simulink library "ITKLib"  (R2022b)
settings: Solver=FixedStepDiscrete  StartTime=0.0  StopTime=10.0  FixedStep=0.01  RelTol=1e-3  EnableMultiTasking=on
values from neighbouring files (symbols this model uses):
  Glb_WhlRollgRd_SC = single(0.36)    [init_Global.m]
undefined symbols (not defined in the file or in its folder): docblock, SlDemoSign, SlDemoSign_Positive_SC, TaskTime_100ms_SC, TaskTime_10ms_SC, VehRefSpd_vMaxRefSpd_C
libraries: simulink x51, $bdroot x45, ITKLib_V14 x1
(part 7 of 10)

== system ITKLib/BitOperation/Subsystem2 ==
  Pos : Inport
  In : Inport  Port=2  OutDataTypeStr=uint8
  Bitwise Operator : simulink/Logic and Bit Operations/Bitwise Operator  logicop=OR  UseBitMask=on  BitMask=bin2dec('00000001')  BitMaskRealWorld=Stored Integer
  Bitwise Operator10 : simulink/Logic and Bit Operations/Bitwise Operator  logicop=OR  UseBitMask=on  BitMask=bin2dec('00100000')  BitMaskRealWorld=Stored Integer
  Bitwise Operator12 : simulink/Logic and Bit Operations/Bitwise Operator  logicop=OR  UseBitMask=on  BitMask=bin2dec('01000000')  BitMaskRealWorld=Stored Integer
  Bitwise Operator14 : simulink/Logic and Bit Operations/Bitwise Operator  logicop=OR  UseBitMask=on  BitMask=bin2dec('10000000')  BitMaskRealWorld=Stored Integer
  Bitwise Operator2 : simulink/Logic and Bit Operations/Bitwise Operator  logicop=OR  UseBitMask=on  BitMask=bin2dec('00000010')  BitMaskRealWorld=Stored Integer
  Bitwise Operator4 : simulink/Logic and Bit Operations/Bitwise Operator  logicop=OR  UseBitMask=on  BitMask=bin2dec('00000100')  BitMaskRealWorld=Stored Integer
  Bitwise Operator6 : simulink/Logic and Bit Operations/Bitwise Operator  logicop=OR  UseBitMask=on  BitMask=bin2dec('00001000')  BitMaskRealWorld=Stored Integer
  Bitwise Operator8 : simulink/Logic and Bit Operations/Bitwise Operator  logicop=OR  UseBitMask=on  BitMask=bin2dec('00010000')  BitMaskRealWorld=Stored Integer
  Multiport Switch : MultiPortSwitch  DataPortOrder=Zero-based contiguous  Inputs=8  DataPortForDefault=Additional data port  DiagnosticForDefault=Warning  zeroidx=on  OutDataTypeStr=uint8  InputSameDT=off
  Out : Outport  VectorParamsAs1DForOutWhenUnconnected=off
  wires:
  Bitwise Operator2/1 -> Multiport Switch/3
  Multiport Switch/1 -> Out/1
  In/1 -> Multiport Switch/10, Bitwise Operator14/1, Bitwise Operator12/1, Bitwise Operator10/1, Bitwise Operator8/1, Bitwise Operator6/1, Bitwise Operator4/1, Bitwise Operator2/1, Bitwise Operator/1
  Bitwise Operator14/1 -> Multiport Switch/9
  Bitwise Operator6/1 -> Multiport Switch/5
  Bitwise Operator8/1 -> Multiport Switch/6
  Bitwise Operator10/1 -> Multiport Switch/7
  Pos/1 -> Multiport Switch/1
  Bitwise Operator4/1 -> Multiport Switch/4
  Bitwise Operator12/1 -> Multiport Switch/8
  Bitwise Operator/1 -> Multiport Switch/2

== system ITKLib/Diagnosis/CheckSum_SGMW ==
  Byte0 : Inport
  Byte1 : Inport  Port=2
  Byte2 : Inport  Port=3
  Byte3 : Inport  Port=4
  Byte4 : Inport  Port=5
  Byte5 : Inport  Port=6
  Byte6 : Inport  Port=7
  CheckSumVal : Inport  Port=8
  Add7 : Sum  Inputs=+++++++  InputSameDT=on  OutDataTypeStr=single  SaturateOnIntegerOverflow=on
  Add8 : Sum  Inputs=+++++++  InputSameDT=on  SaturateOnIntegerOverflow=on
  DataTypeConversion1 : DataTypeConversion  OutDataTypeStr=single  SaturateOnIntegerOverflow=off  RndMeth=Floor
  DataTypeConversion{2,9..10,21} (4 alike) : DataTypeConversion  OutDataTypeStr=uint8  SaturateOnIntegerOverflow=off  RndMeth=Floor
  DataTypeConversion20 : DataTypeConversion  OutDataTypeStr=single  SaturateOnIntegerOverflow=off
  DataTypeConversion3 : DataTypeConversion  OutDataTypeStr=single  SaturateOnIntegerOverflow=off  RndMeth=Floor
  DataTypeConversion4 : DataTypeConversion  OutDataTypeStr=uint8  SaturateOnIntegerOverflow=off
  DataTypeConversion5 : DataTypeConversion  OutDataTypeStr=single  SaturateOnIntegerOverflow=off  RndMeth=Floor
  Demux4 : Demux  Outputs=7
  Equal3 : RelationalOperator  Operator=~=  OutDataTypeStr=boolean
  Minus : Sum  Inputs=+-  InputSameDT=on  SaturateOnIntegerOverflow=on
  Minus1 : Sum  InputSameDT=on  SaturateOnIntegerOverflow=on
  Minus2 : Sum  Inputs=+-  InputSameDT=on  SaturateOnIntegerOverflow=on
  Mux4 : Mux  Inputs=7
  Product1 : Product  Inputs=*/  InputSameDT=on  SaturateOnIntegerOverflow=on
  Product2 : Product  Inputs=*/  InputSameDT=on  SaturateOnIntegerOverflow=on
  Product3 : Product  InputSameDT=on  SaturateOnIntegerOverflow=on
  Product4 : Product  Inputs=*/  InputSameDT=on  SaturateOnIntegerOverflow=on
  Product5 : Product  InputSameDT=on  SaturateOnIntegerOverflow=on
  Product6 : Product  InputSameDT=on  SaturateOnIntegerOverflow=on
  single33 : Constant  Value=16  OutDataTypeStr=uint8
      settings: AttributesFormatString=%<OutDataTypeStr>
  single40 : Constant  Value=16  OutDataTypeStr=single
      settings: AttributesFormatString=%<OutDataTypeStr>
  single41 : Constant  Value=16  OutDataTypeStr=single
      settings: AttributesFormatString=%<OutDataTypeStr>
  single50 : Constant  Value=16  OutDataTypeStr=single
      settings: AttributesFormatString=%<OutDataTypeStr>
  CheckSumErr : Outport
  CheckSumCalc : Outport  Port=2
  wires:
  Product1/1 -> DataTypeConversion21/1
  Byte0/1 -> Mux4/1, Add7/1
  single50/1 -> Product6/2, Product1/2
  Byte3/1 -> Mux4/4, Add7/4
  Product6/1 -> Minus2/2
  Byte2/1 -> Mux4/3, Add7/3
  CheckSumVal/1 -> DataTypeConversion9/1
  single40/1 -> Product5/2
  Product5/1 -> Minus1/2
  DataTypeConversion9/1 -> Equal3/2
  DataTypeConversion10/1 -> DataTypeConversion5/1
  Equal3/1 -> CheckSumErr/1
  single33/1 -> Product4/2
  Minus1/1 -> CheckSumCalc/1, DataTypeConversion4/1
  Demux4/4 -> Add8/4
  Demux4/6 -> Add8/6
  Demux4/1 -> Add8/1
  Demux4/5 -> Add8/5
  Add7/1 -> DataTypeConversion1/1
  Demux4/2 -> Add8/2
  Demux4/3 -> Add8/3
  Byte6/1 -> Mux4/7, Add7/7
  Add8/1 -> DataTypeConversion20/1
  Product4/1 -> Demux4/1
  Product3/1 -> Minus/2
  Product2/1 -> DataTypeConversion10/1
  Demux4/7 -> Add8/7
  Byte4/1 -> Mux4/5, Add7/5
  Mux4/1 -> DataTypeConversion2/1
  Byte1/1 -> Mux4/2, Add7/2
  Byte5/1 -> Mux4/6, Add7/6
  DataTypeConversion2/1 -> Product4/1
  single41/1 -> Product3/2, Product2/2
  DataTypeConversion20/1 -> Minus2/1, Product1/1
  Minus2/1 -> Product5/1
  DataTypeConversion1/1 -> Minus/1, Product2/1
  DataTypeConversion5/1 -> Product3/1
  Minus/1 -> Minus1/1
  DataTypeConversion21/1 -> DataTypeConversion3/1
  DataTypeConversion3/1 -> Product6/1
  DataTypeConversion4/1 -> Equal3/1

== system ITKLib/Diagnosis/Debounce_OBD ==
  bErr : Inport  OutDataTypeStr=boolean
  bRst : Inport  Port=2  OutDataTypeStr=boolean
  bEna : Inport  Port=3  OutDataTypeStr=boolean  PortDimensions=1
  FailThd : Inport  Port=4  OutDataTypeStr=int16
  RecThd : Inport  Port=5  OutDataTypeStr=int16
  IncrFail : Inport  Port=6  OutDataTypeStr=int16
  DecrRec : Inport  Port=7  OutDataTypeStr=int16
  DebounceEnable : Subsystem
  Debounce_OBD : Subsystem  TreatAsAtomicUnit=on
  Unit Delay1 : UnitDelay  SampleTime=-1  HasFrameUpgradeWarning=on
      settings: AttributesFormatString=<initial=%<X0>>
  Unit Delay2 : UnitDelay  SampleTime=-1  HasFrameUpgradeWarning=on
      settings: AttributesFormatString=<initial=%<X0>>
  bFailed : Outport
  wires:
  DecrRec/1 -> Debounce_OBD/6(DecrRec)
  IncrFail/1 -> Debounce_OBD/5(IncrFail)
  Debounce_OBD/2(bFailed) -> Unit Delay1/1, bFailed/1
  bErr/1 -> DebounceEnable/5(bErr), Debounce_OBD/1(bErr)
  bRst/1 -> Debounce_OBD/2(bRst), DebounceEnable/4(bRst)
  FailThd/1 -> Debounce_OBD/3(FailThd)
  RecThd/1 -> Debounce_OBD/4(RecThd)
  bEna/1 -> DebounceEnable/3(bEna)
  Debounce_OBD/1(bOutRanged) -> Unit Delay2/1
  DebounceEnable/1(bDebounceEna) -> Debounce_OBD/Enable
  Unit Delay2/1 -> DebounceEnable/1(bOutRangedOld)
  Unit Delay1/1 -> DebounceEnable/2(bFailedOld)

== system ITKLib/Diagnosis/FltCollctn ==
  FltFlg : Inport
  FltNr : Inport  Port=2
  FltPos : Subsystem
  FltStAry : Stateflow chart  TreatAsAtomicUnit=on
  FltStCodAry : Stateflow chart  TreatAsAtomicUnit=on
  wires:
  FltPos/2(BitPos) -> FltStCodAry/3(BitPos)
  FltFlg/1 -> FltStAry/2(FltFlg), FltStCodAry/1(FltFlg)
  FltNr/1 -> FltPos/1(FltNr), FltStAry/1(FltNr)
  FltPos/1(AryIdx) -> FltStCodAry/2(AryIdx)

== system ITKLib/Diagnosis/FltLatchCollctn ==
  FltFlg : Inport
  SentCod : Inport  Port=2
  FltNr : Inport  Port=3
  FltPos : Subsystem
  FltStAry : Stateflow chart  TreatAsAtomicUnit=on
  FltStCodAry : Stateflow chart  TreatAsAtomicUnit=on
  Max : MinMax  Function=max  Inputs=2  InputSameDT=on  SaturateOnIntegerOverflow=on
  Subsystem : Subsystem
  uint8 : Constant  OutDataTypeStr=uint8  SampleTime=-1
      settings: AttributesFormatString=%<OutDataTypeStr>
  wires:
  FltPos/1(AryIdx) -> FltStCodAry/2(AryIdx)
  FltPos/2(BitPos) -> FltStCodAry/3(BitPos)
  Max/1 -> FltPos/1(FltNr), FltStAry/1(FltNr), Subsystem/1(FltNr)
  Subsystem/1(FltFlg1) -> FltStCodAry/1(FltFlg), FltStAry/2(FltFlg)
  FltFlg/1 -> Subsystem/2(FltFlg)
  SentCod/1 -> Subsystem/3(SentCod)
  FltNr/1 -> Max/1
  uint8/1 -> Max/2

== system ITKLib/Diagnosis/FltMux ==
  FltFlg : Inport  OutDataTypeStr=boolean
  FltOpenEna : Inport  Port=2  OutDataTypeStr=boolean
  SentCod : Inport  Port=3
  AND : Logic  OutDataTypeStr=boolean
  Bus Creator : BusCreator  Inputs=5
  Constant1 : Constant  Value=FltCod  OutDataTypeStr=uint8
  Constant15 : Constant  Value=TqRdcFac  OutDataTypeStr=uint8
  Constant2 : Constant  Value=FltCod  OutDataTypeStr=uint8
  Constant29 : Constant  Value=MaiFltLvl  OutMax=10  OutDataTypeStr=uint8
  Constant5 : Constant  Value=SubFltLvl  OutMax=3  OutDataTypeStr=uint8
  Constant6 : Constant  Value=TqRdcEna  OutDataTypeStr=boolean
  Constant8 : Constant  Value=ClsIgbtEna  OutDataTypeStr=boolean
  Demux : Demux
  Equal{,1..3} (4 alike) : RelationalOperator  Operator===  OutDataTypeStr=boolean  RndMeth=Simplest  InputSameDT=off
  Logical Operator : Logic  OutDataTypeStr=boolean
  Logical Operator3 : Logic  OutDataTypeStr=boolean
  Logical Operator4 : Logic  OutDataTypeStr=boolean
  Not : Logic  Operator=NOT  AllPortsSameDT=off  OutDataTypeStr=boolean
  OR : Logic  Operator=OR  Inputs=4  OutDataTypeStr=boolean
  Product : Product  InputSameDT=on  SaturateOnIntegerOverflow=on
  RSLatch : $bdroot/Memory/RSLatch
  Relational Operator2 : RelationalOperator  OutDataTypeStr=boolean
  Switch{2,4..7} (5 alike) : Switch  Criteria=u2 ~= 0  SaturateOnIntegerOverflow=off  InputSameDT=off
      settings: AttributesFormatString=Criteria : %<Criteria>
  single : Constant  Value=100  OutDataTypeStr=single  SampleTime=-1
      settings: AttributesFormatString=%<OutDataTypeStr>
  single1 : Constant  Value=0.01  OutDataTypeStr=single  SampleTime=-1
      settings: AttributesFormatString=%<OutDataTypeStr>
  uint16 : Constant  Value=0  OutDataTypeStr=uint16  SampleTime=-1
      settings: AttributesFormatString=%<OutDataTypeStr>
  uint3 : Constant  Value=0  OutDataTypeStr=uint8  SampleTime=-1
      settings: AttributesFormatString=%<OutDataTypeStr>
  uint4 : Constant  Value=3  OutDataTypeStr=uint8  SampleTime=-1
      settings: AttributesFormatString=%<OutDataTypeStr>
  uint5 : Constant  Value=3  OutDataTypeStr=uint8  SampleTime=-1
      settings: AttributesFormatString=%<OutDataTypeStr>
  uint6 : Constant  Value=0  OutDataTypeStr=uint8  SampleTime=-1
      settings: AttributesFormatString=%<OutDataTypeStr>
  FltMux : Outport  VectorParamsAs1DForOutWhenUnconnected=off
  wires:
  uint6/1 -> Switch7/3
  Switch5/1 -> Bus Creator/1  "MaiFltLvl"
  uint3/1 -> Switch5/3
  Constant5/1 -> Relational Operator2/1, Switch6/3
  FltFlg/1 -> Logical Operator/1
  Product/1 -> Bus Creator/5  "TqRdcFac"
  Logical Operator4/1 -> Bus Creator/4  "ClsIgbtActv"
  Constant29/1 -> Switch5/1
  Constant2/1 -> Switch2/1
  Constant8/1 -> Logical Operator4/2
  Switch2/1 -> Bus Creator/3  "FltCod"
  Switch6/1 -> Switch7/1
  uint16/1 -> Switch2/3
  uint5/1 -> Switch6/1
  single/1 -> Switch4/3
  Logical Operator3/1 -> Switch4/2
  Constant6/1 -> Logical Operator3/2
  Constant15/1 -> Switch4/1
  Relational Operator2/1 -> Switch6/2
  Switch7/1 -> Bus Creator/2  "SubFltLvl"
  Bus Creator/1 -> FltMux/1
  FltOpenEna/1 -> Logical Operator/2
  uint4/1 -> Relational Operator2/2
  Switch4/1 -> Product/1
  single1/1 -> Product/2
  Equal3/1 -> OR/4
  AND/1 -> RSLatch/2
  Demux/1 -> Equal/1
  Demux/2 -> Equal1/1
  Logical Operator/1 -> Switch7/2, RSLatch/1, Logical Operator3/1, Logical Operator4/1, Not/1, Switch5/2
  OR/1 -> AND/1
  Demux/4 -> Equal3/1
  Equal1/1 -> OR/2
  Equal/1 -> OR/1
  SentCod/1 -> Demux/1
  Constant1/1 -> Equal1/2, Equal/2, Equal2/2, Equal3/2
  Not/1 -> AND/2
  Equal2/1 -> OR/3
  Demux/3 -> Equal2/1
  RSLatch/1 -> Switch2/2

== system ITKLib/Diagnosis/LifeCycleCounter ==
  MaxCnt : Inport
  Add : Sum
  Equal : RelationalOperator  OutDataTypeStr=boolean  RndMeth=Simplest  InputSameDT=off
  FALSE : Constant  Description=FALSE  Value=0  OutDataTypeStr=boolean
      settings: AttributesFormatString=%<Description>
  Saturation2 : Saturate  UpperLimit=uint16(65534)  LowerLimit=uint16(0)
      settings: AttributesFormatString=|
      | UpperLimit = %<UpperLimit>
      | LowLimit = %<LowerLimit>
  Switch : Switch  Criteria=u2 ~= 0  SaturateOnIntegerOverflow=off  InputSameDT=off
      settings: AttributesFormatString=Criteria : %<Criteria>
  Switch1 : Switch  Criteria=u2 ~= 0  SaturateOnIntegerOverflow=off  InputSameDT=off
      settings: AttributesFormatString=Criteria : %<Criteria>
  TRUE : Constant  Description=TRUE  OutDataTypeStr=boolean
      settings: AttributesFormatString=%<Description>
  Unit Delay2 : UnitDelay  SampleTime=-1  HasFrameUpgradeWarning=on
      settings: AttributesFormatString=<initial=%<x0>>
  Unit Delay5 : UnitDelay  InitialCondition=uint16(0)  SampleTime=-1  HasFrameUpgradeWarning=on
      settings: AttributesFormatString=<initial=%<x0>>
  uint2 : Constant  OutDataTypeStr=uint16
      settings: AttributesFormatString=%<OutDataTypeStr>
  uint8 : Constant  Value=0  OutDataTypeStr=uint16
      settings: AttributesFormatString=%<OutDataTypeStr>
  LifeCycleCnt : Outport
  wires:
  FALSE/1 -> Switch1/1
  TRUE/1 -> Switch1/3
  Switch1/1 -> Unit Delay2/1
  Add/1 -> Switch/1
  MaxCnt/1 -> Equal/2
  uint8/1 -> Switch/3
  Switch/1 -> Saturation2/1
  uint2/1 -> Add/2
  Unit Delay5/1 -> Add/1
  Unit Delay2/1 -> Switch/2
  Equal/1 -> Switch1/2
  Saturation2/1 -> Unit Delay5/1, Equal/1, LifeCycleCnt/1

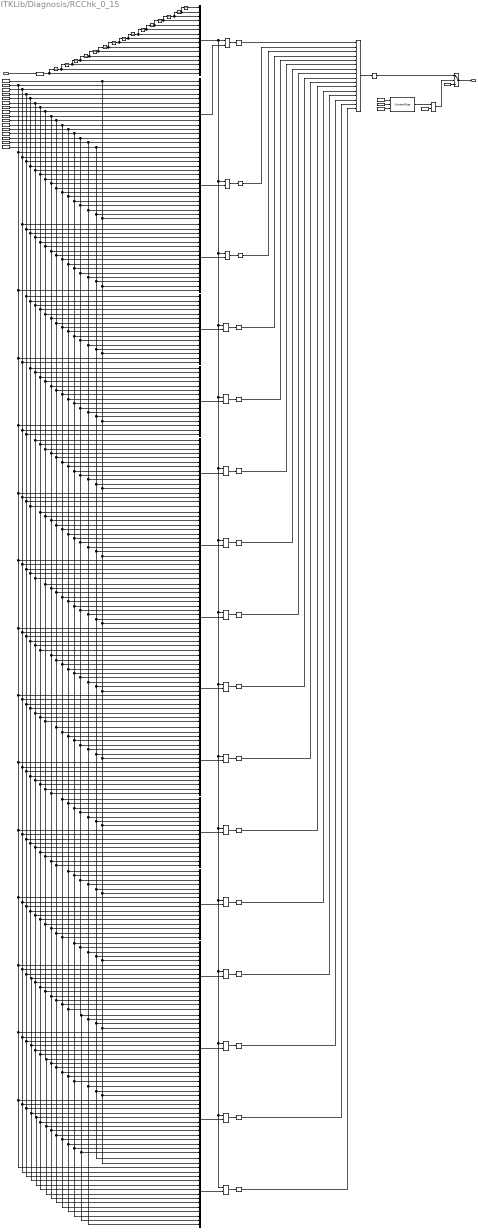
== system ITKLib/Diagnosis/RCChk_0_15 ==
  In : Inport
  AND{4..19} (16 alike) : Logic  Inputs=1  OutDataTypeStr=boolean
  CounterRStep : $bdroot/TimeCounter/CounterRStep  Cnt_Max=uint16(400)
      settings: AttributesFormatString=|
      | CounterRStep
      | Cnt_Max=%<Cnt_Max>
  DataTypeConversion1 : DataTypeConversion  OutDataTypeStr=uint8  SaturateOnIntegerOverflow=off  RndMeth=Floor
  Equal{5..20} (16 alike) : RelationalOperator  Operator===  OutDataTypeStr=boolean
  FALSE : Constant  Description=FALSE  Value=0  OutDataTypeStr=boolean  SampleTime=-1
      settings: AttributesFormatString=%<Description>
  FALSE1 : Constant  Description=FALSE  Value=0  OutDataTypeStr=boolean  SampleTime=-1
      settings: AttributesFormatString=%<Description>
  GreaterOrEqual : RelationalOperator  Operator=>  OutDataTypeStr=boolean
  Logical Operator9 : Logic  Operator=NOT  AllPortsSameDT=off  OutDataTypeStr=boolean
  Mux{5..21} (17 alike) : Mux  Inputs=16
  OR1 : Logic  Operator=OR  Inputs=16  OutDataTypeStr=boolean
  Switch : Switch  Criteria=u2 ~= 0  SaturateOnIntegerOverflow=off  InputSameDT=off
      settings: AttributesFormatString=Criteria : %<Criteria>
  TRUE : Constant  Description=TRUE  OutDataTypeStr=boolean  SampleTime=-1
      settings: AttributesFormatString=%<Description>
  UnitDelay{1..15} (15 alike) : UnitDelay  SampleTime=-1  HasFrameUpgradeWarning=on
      settings: AttributesFormatString=<Initial=%<x0>>
  uint1 : Constant  OutDataTypeStr=uint16  SampleTime=-1
      settings: AttributesFormatString=%<OutDataTypeStr>
  uint17 : Constant  OutDataTypeStr=uint8
      settings: AttributesFormatString=%<OutDataTypeStr>
  uint18 : Constant  Value=16  OutDataTypeStr=uint16  SampleTime=-1
      settings: AttributesFormatString=%<OutDataTypeStr>
  uint25 : Constant  Value=2  OutDataTypeStr=uint8
      settings: AttributesFormatString=%<OutDataTypeStr>
  uint26 : Constant  Value=3  OutDataTypeStr=uint8
      settings: AttributesFormatString=%<OutDataTypeStr>
  uint31 : Constant  Value=0  OutDataTypeStr=uint8
      settings: AttributesFormatString=%<OutDataTypeStr>
  uint33 : Constant  Value=4  OutDataTypeStr=uint8
      settings: AttributesFormatString=%<OutDataTypeStr>
  uint34 : Constant  Value=5  OutDataTypeStr=uint8
      settings: AttributesFormatString=%<OutDataTypeStr>
  uint35 : Constant  Value=6  OutDataTypeStr=uint8
      settings: AttributesFormatString=%<OutDataTypeStr>
  uint36 : Constant  Value=7  OutDataTypeStr=uint8
      settings: AttributesFormatString=%<OutDataTypeStr>
  uint37 : Constant  Value=8  OutDataTypeStr=uint8
      settings: AttributesFormatString=%<OutDataTypeStr>
  uint38 : Constant  Value=9  OutDataTypeStr=uint8
      settings: AttributesFormatString=%<OutDataTypeStr>
  uint39 : Constant  Value=10  OutDataTypeStr=uint8
      settings: AttributesFormatString=%<OutDataTypeStr>
  uint40 : Constant  Value=11  OutDataTypeStr=uint8
      settings: AttributesFormatString=%<OutDataTypeStr>
  uint41 : Constant  Value=12  OutDataTypeStr=uint8
      settings: AttributesFormatString=%<OutDataTypeStr>
  uint42 : Constant  Value=13  OutDataTypeStr=uint8
      settings: AttributesFormatString=%<OutDataTypeStr>
  uint43 : Constant  Value=14  OutDataTypeStr=uint8
      settings: AttributesFormatString=%<OutDataTypeStr>
  uint44 : Constant  Value=15  OutDataTypeStr=uint8
      settings: AttributesFormatString=%<OutDataTypeStr>
  RCErr : Outport
  wires:
  Logical Operator9/1 -> Switch/1
  OR1/1 -> Logical Operator9/1
  Equal12/1 -> AND11/1
  uint37/1 -> Mux21/10, Mux20/11, Mux19/12, Mux18/13, Mux17/14, Mux16/15, Mux15/16, Mux14/1, Mux13/2, Mux12/3, Mux11/4, Mux10/5, Mux9/6, Mux8/7, Mux7/8, Mux6/9
  AND19/1 -> OR1/16
  Mux11/1 -> Equal10/2
  AND17/1 -> OR1/14
  Equal18/1 -> AND17/1
  UnitDelay7/1 -> UnitDelay8/1, Mux5/11
  AND18/1 -> OR1/15
  UnitDelay4/1 -> UnitDelay5/1, Mux5/14
  AND16/1 -> OR1/13
  AND13/1 -> OR1/10
  AND15/1 -> OR1/12
  UnitDelay12/1 -> UnitDelay13/1, Mux5/6
  Mux20/1 -> Equal19/2
  AND10/1 -> OR1/7
  Equal5/1 -> AND4/1
  uint35/1 -> Mux19/10, Mux21/8, Mux20/9, Mux18/11, Mux17/12, Mux16/13, Mux15/14, Mux14/15, Mux13/16, Mux12/1, Mux11/2, Mux10/3, Mux9/4, Mux8/5, Mux7/6, Mux6/7
  UnitDelay5/1 -> UnitDelay6/1, Mux5/13
  Equal16/1 -> AND15/1
  UnitDelay10/1 -> UnitDelay11/1, Mux5/8
  uint36/1 -> Mux21/9, Mux20/10, Mux19/11, Mux18/12, Mux17/13, Mux16/14, Mux15/15, Mux14/16, Mux13/1, Mux12/2, Mux11/3, Mux10/4, Mux9/5, Mux8/6, Mux7/7, Mux6/8
  Mux21/1 -> Equal20/2
  uint17/1 -> Mux21/3, Mux20/4, Mux19/5, Mux18/6, Mux17/7, Mux16/8, Mux15/9, Mux14/10, Mux13/11, Mux12/12, Mux11/13, Mux10/14, Mux9/15, Mux8/16, Mux7/1, Mux6/2
  Mux16/1 -> Equal15/2
  Equal19/1 -> AND18/1
  Mux14/1 -> Equal13/2
  Mux15/1 -> Equal14/2
  Equal14/1 -> AND13/1
  Equal17/1 -> AND16/1
  Mux18/1 -> Equal17/2
  uint25/1 -> Mux9/16, Mux21/4, Mux20/5, Mux19/6, Mux18/7, Mux17/8, Mux16/9, Mux15/10, Mux14/11, Mux13/12, Mux12/13, Mux11/14, Mux10/15, Mux8/1, Mux7/2, Mux6/3
  Equal15/1 -> AND14/1
  AND7/1 -> OR1/4
  Equal10/1 -> AND9/1
  uint43/1 -> Mux21/16, Mux20/1, Mux19/2, Mux18/3, Mux17/4, Mux16/5, Mux15/6, Mux14/7, Mux13/8, Mux12/9, Mux11/10, Mux10/11, Mux9/12, Mux8/13, Mux7/14, Mux6/15
  Mux19/1 -> Equal18/2
  AND9/1 -> OR1/6
  Equal20/1 -> AND19/1
  Mux17/1 -> Equal16/2
  Equal13/1 -> AND12/1
  AND11/1 -> OR1/8
  Mux7/1 -> Equal6/2
  uint40/1 -> Mux21/13, Mux20/14, Mux19/15, Mux18/16, Mux17/1, Mux16/2, Mux15/3, Mux14/4, Mux13/5, Mux12/6, Mux11/7, Mux10/8, Mux9/9, Mux8/10, Mux7/11, Mux6/12
  uint38/1 -> Mux21/11, Mux20/12, Mux19/13, Mux18/14, Mux17/15, Mux16/16, Mux15/1, Mux14/2, Mux13/3, Mux12/4, Mux11/5, Mux10/6, Mux9/7, Mux8/8, Mux7/9, Mux6/10
  Mux9/1 -> Equal8/2
  uint42/1 -> Mux21/15, Mux20/16, Mux19/1, Mux18/2, Mux17/3, Mux16/4, Mux15/5, Mux14/6, Mux13/7, Mux12/8, Mux11/9, Mux10/10, Mux9/11, Mux8/12, Mux7/13, Mux6/14
  UnitDelay1/1 -> UnitDelay2/1, Mux5/2
  Mux5/1 -> Equal20/1, Equal19/1, Equal18/1, Equal17/1, Equal16/1, Equal15/1, Equal14/1, Equal13/1, Equal12/1, Equal11/1, Equal10/1, Equal9/1, Equal8/1, Equal7/1, Equal6/1, Equal5/1
  UnitDelay2/1 -> Mux5/1
  uint41/1 -> Mux21/14, Mux20/15, Mux19/16, Mux18/1, Mux17/2, Mux16/3, Mux15/4, Mux14/5, Mux13/6, Mux12/7, Mux11/8, Mux10/9, Mux9/10, Mux8/11, Mux7/12, Mux6/13
  Mux6/1 -> Equal5/2
  Mux10/1 -> Equal9/2
  Mux13/1 -> Equal12/2
  uint44/1 -> Mux21/1, Mux20/2, Mux19/3, Mux18/4, Mux17/5, Mux16/6, Mux15/7, Mux14/8, Mux13/9, Mux12/10, Mux11/11, Mux10/12, Mux9/13, Mux8/14, Mux7/15, Mux6/16
  UnitDelay9/1 -> UnitDelay10/1, Mux5/9
  UnitDelay14/1 -> UnitDelay15/1, Mux5/4
  UnitDelay11/1 -> UnitDelay12/1, Mux5/7
  uint31/1 -> Mux21/2, Mux20/3, Mux19/4, Mux18/5, Mux17/6, Mux16/7, Mux15/8, Mux14/9, Mux13/10, Mux12/11, Mux11/12, Mux10/13, Mux9/14, Mux8/15, Mux7/16, Mux6/1
  UnitDelay13/1 -> UnitDelay14/1, Mux5/5
  uint39/1 -> Mux21/12, Mux20/13, Mux19/14, Mux18/15, Mux17/16, Mux16/1, Mux15/2, Mux14/3, Mux13/4, Mux12/5, Mux11/6, Mux10/7, Mux9/8, Mux8/9, Mux7/10, Mux6/11
  uint26/1 -> Mux21/5, Mux20/6, Mux19/7, Mux18/8, Mux17/9, Mux16/10, Mux15/11, Mux14/12, Mux13/13, Mux12/14, Mux11/15, Mux10/16, Mux9/1, Mux8/2, Mux7/3, Mux6/4
  Equal11/1 -> AND10/1
  Mux12/1 -> Equal11/2
  UnitDelay8/1 -> UnitDelay9/1, Mux5/10
  uint34/1 -> Mux21/7, Mux20/8, Mux19/9, Mux18/10, Mux17/11, Mux16/12, Mux15/13, Mux14/14, Mux13/15, Mux12/16, Mux11/1, Mux10/2, Mux9/3, Mux8/4, Mux7/5, Mux6/6
  AND8/1 -> OR1/5
  DataTypeConversion1/1 -> Mux5/16, UnitDelay3/1
  AND4/1 -> OR1/1
  AND6/1 -> OR1/3
  Equal7/1 -> AND6/1
  AND5/1 -> OR1/2
  uint33/1 -> Mux21/6, Mux20/7, Mux19/8, Mux18/9, Mux17/10, Mux16/11, Mux15/12, Mux14/13, Mux13/14, Mux12/15, Mux11/16, Mux10/1, Mux9/2, Mux8/3, Mux7/4, Mux6/5
  Equal8/1 -> AND7/1
  UnitDelay3/1 -> UnitDelay4/1, Mux5/15
  AND12/1 -> OR1/9
  Equal6/1 -> AND5/1
  UnitDelay15/1 -> UnitDelay1/1, Mux5/3
  Mux8/1 -> Equal7/2
  Equal9/1 -> AND8/1
  AND14/1 -> OR1/11
  UnitDelay6/1 -> UnitDelay7/1, Mux5/12
  In/1 -> DataTypeConversion1/1
  CounterRStep/1 -> GreaterOrEqual/1
  FALSE/1 -> CounterRStep/2
  uint18/1 -> GreaterOrEqual/2
  TRUE/1 -> CounterRStep/1
  FALSE1/1 -> Switch/3
  uint1/1 -> CounterRStep/3
  GreaterOrEqual/1 -> Switch/2
  Switch/1 -> RCErr/1

== system ITKLib/Diagnosis/RCChk_0_3 ==
  In : Inport
  AND{,1..3} (4 alike) : Logic  Inputs=1  OutDataTypeStr=boolean
  CounterRStep : $bdroot/TimeCounter/CounterRStep  Cnt_Max=uint16(400)
      settings: AttributesFormatString=|
      | CounterRStep
      | Cnt_Max=%<Cnt_Max>
  DataTypeConversion : DataTypeConversion  OutDataTypeStr=uint8  SaturateOnIntegerOverflow=off  RndMeth=Floor
  Equal{1..4} (4 alike) : RelationalOperator  Operator===  OutDataTypeStr=boolean
  FALSE : Constant  Description=FALSE  Value=0  OutDataTypeStr=boolean  SampleTime=-1
      settings: AttributesFormatString=%<Description>
  FALSE1 : Constant  Description=FALSE  Value=0  OutDataTypeStr=boolean  SampleTime=-1
      settings: AttributesFormatString=%<Description>
  GreaterOrEqual : RelationalOperator  Operator=>  OutDataTypeStr=boolean
  Logical Operator9 : Logic  Operator=NOT  AllPortsSameDT=off  OutDataTypeStr=boolean
  Mux{,1..4} (5 alike) : Mux
  OR : Logic  Operator=OR  Inputs=4  OutDataTypeStr=boolean
  Switch : Switch  Criteria=u2 ~= 0  SaturateOnIntegerOverflow=off  InputSameDT=off
      settings: AttributesFormatString=Criteria : %<Criteria>
  TRUE : Constant  Description=TRUE  OutDataTypeStr=boolean  SampleTime=-1
      settings: AttributesFormatString=%<Description>
  UnitDelay : UnitDelay  SampleTime=-1  HasFrameUpgradeWarning=on
      settings: AttributesFormatString=<Initial=%<x0>>
  UnitDelay1 : UnitDelay  SampleTime=-1  HasFrameUpgradeWarning=on
      settings: AttributesFormatString=<Initial=%<x0>>
  UnitDelay2 : UnitDelay  SampleTime=-1  HasFrameUpgradeWarning=on
      settings: AttributesFormatString=<Initial=%<x0>>
  uint{1,4,12,14} (4 alike) : Constant  OutDataTypeStr=uint8
      settings: AttributesFormatString=%<OutDataTypeStr>
  uint{2,5,10,16} (4 alike) : Constant  Value=2  OutDataTypeStr=uint8
      settings: AttributesFormatString=%<OutDataTypeStr>
  uint{3,6,11,13} (4 alike) : Constant  Value=3  OutDataTypeStr=uint8
      settings: AttributesFormatString=%<OutDataTypeStr>
  uint{7..9,15} (4 alike) : Constant  Value=0  OutDataTypeStr=uint8
      settings: AttributesFormatString=%<OutDataTypeStr>
  uint17 : Constant  OutDataTypeStr=uint16  SampleTime=-1
      settings: AttributesFormatString=%<OutDataTypeStr>
  uint18 : Constant  Value=4  OutDataTypeStr=uint16  SampleTime=-1
      settings: AttributesFormatString=%<OutDataTypeStr>
  RCErr : Outport
  wires:
  Mux4/1 -> Equal4/2
  UnitDelay2/1 -> Mux/1
  DataTypeConversion/1 -> Mux/4, UnitDelay/1
  uint8/1 -> Mux1/1
  OR/1 -> Logical Operator9/1
  uint1/1 -> Mux1/2
  Mux/1 -> Equal1/1, Equal2/1, Equal3/1, Equal4/1
  uint16/1 -> Mux4/4
  AND3/1 -> OR/4
  Equal2/1 -> AND1/1
  uint10/1 -> Mux3/1
  uint2/1 -> Mux1/3
  Logical Operator9/1 -> Switch/1
  uint13/1 -> Mux4/1
  uint7/1 -> Mux2/4
  UnitDelay1/1 -> UnitDelay2/1, Mux/2
  Mux2/1 -> Equal2/2
  Mux3/1 -> Equal3/2
  Mux1/1 -> Equal1/2
  uint15/1 -> Mux4/2
  uint14/1 -> Mux4/3
  Equal1/1 -> AND/1
  uint9/1 -> Mux3/3
  Equal4/1 -> AND3/1
  uint11/1 -> Mux3/2
  uint5/1 -> Mux2/2
  AND1/1 -> OR/2
  uint12/1 -> Mux3/4
  uint4/1 -> Mux2/1
  uint3/1 -> Mux1/4
  uint6/1 -> Mux2/3
  In/1 -> DataTypeConversion/1
  AND2/1 -> OR/3
  Equal3/1 -> AND2/1
  UnitDelay/1 -> Mux/3, UnitDelay1/1
  AND/1 -> OR/1
  TRUE/1 -> CounterRStep/1
  FALSE/1 -> CounterRStep/2
  uint17/1 -> CounterRStep/3
  CounterRStep/1 -> GreaterOrEqual/1
  uint18/1 -> GreaterOrEqual/2
  GreaterOrEqual/1 -> Switch/2
  FALSE1/1 -> Switch/3
  Switch/1 -> RCErr/1

== system ITKLib/Diagnosis/RollgCntrChk ==
  RollgCntr : Inport  OutDataTypeStr=uint8
  RollgCntrMax : Inport  Port=2  OutDataTypeStr=uint8
  RollgCntrErrThd : Inport  Port=3  OutDataTypeStr=uint8
  Add : Sum  InputSameDT=on  SaturateOnIntegerOverflow=on
  DataTypeConversion : DataTypeConversion  OutDataTypeStr=uint16  RndMeth=Nearest  SaturateOnIntegerOverflow=off
  DataTypeConversion1 : DataTypeConversion  OutDataTypeStr=uint16  RndMeth=Nearest  SaturateOnIntegerOverflow=off
  DataTypeConversion2 : DataTypeConversion  OutDataTypeStr=uint16  RndMeth=Nearest  SaturateOnIntegerOverflow=off
  Equal1 : RelationalOperator  Operator===  OutDataTypeStr=boolean
  Equal2 : RelationalOperator  Operator=~=  OutDataTypeStr=boolean
  Equal3 : RelationalOperator  Operator===  OutDataTypeStr=boolean
  Equal4 : RelationalOperator  Operator=~=  OutDataTypeStr=boolean
  Greater : RelationalOperator  Operator=>  OutDataTypeStr=boolean
  GreaterOrEqual1 : RelationalOperator  OutDataTypeStr=boolean
  Logical Operator1 : Logic  Operator=NOT  AllPortsSameDT=off  OutDataTypeStr=boolean
  OR : Logic  Operator=OR  OutDataTypeStr=boolean
  RSLatch : Subsystem  RTWFcnName=RS_Latch  RTWFileName=ITK_Mdl_Lib  mask(RSLatch){}
      mask help:
      | RS latch with initial value
      | Set signal is passed from port 'S'
      | Reset signal is passed from port 'R'
      | Initial value is passed from port 'IV'
      |
      | Q is set if S is set and reset if R is set.
      | The reset logic is of higher priority than set logic.
      | The initial state is set by IV.
      |
      | Simulink Custom Model Library, created by MCC.
      mask Help:
      | RS latch with initial value
      | Set signal is passed from port 'S'
      | Reset signal is passed from port 'R'
      | Initial value is passed from port 'IV'
      | 
      | Q is set if S is set and reset if R is set.
      | The reset logic is of higher priority than set logic.
      | The initial state is set by IV.
      mask Display:
      | color('blue')
      | disp('\fontsize{12}RS Latch', 'texmode', 'on')
      | color('black');
      | port_label('input', 1, 'S', 'texmode', 'on')
      | port_label('input', 2, 'R', 'texmode', 'on')
      | port_label('output', 1, 'Q', 'texmode', 'on')
      | color('green');
      | text(1,0,'ITK','horizontalAlignment','right','verticalAlignment','bottom');
  Subtract : Sum  Inputs=+-  InputSameDT=on
  Switch1 : Switch  Criteria=u2 ~= 0  SaturateOnIntegerOverflow=off  InputSameDT=off
      settings: AttributesFormatString=Criteria : %<Criteria>
  Switch3 : Switch  Criteria=u2 ~= 0  SaturateOnIntegerOverflow=off  InputSameDT=off
      settings: AttributesFormatString=Criteria : %<Criteria>
  Unit Delay : UnitDelay  SampleTime=-1  HasFrameUpgradeWarning=on
      settings: AttributesFormatString=<initial=%<x0>>
  UnitDelay3 : UnitDelay  SampleTime=-1  HasFrameUpgradeWarning=on
      settings: AttributesFormatString=<Initial=%<x0>>
  uint2 : Constant  Value=0  OutDataTypeStr=uint16  SampleTime=-1
      settings: AttributesFormatString=%<OutDataTypeStr>
  uint4 : Constant  OutDataTypeStr=uint16  SampleTime=-1
      settings: AttributesFormatString=%<OutDataTypeStr>
  uint6 : Constant  Value=0  OutDataTypeStr=uint16  SampleTime=-1
      settings: AttributesFormatString=%<OutDataTypeStr>
  uint8 : Constant  OutDataTypeStr=uint16  SampleTime=-1
      settings: AttributesFormatString=%<OutDataTypeStr>
  RollgCntrErr : Outport
  wires:
  OR/1 -> RollgCntrErr/1
  DataTypeConversion/1 -> UnitDelay3/1, Subtract/1, Equal1/1, Greater/1, Equal4/1
  RollgCntrMax/1 -> DataTypeConversion1/1
  Greater/1 -> OR/2
  Equal1/1 -> Logical Operator1/1
  uint8/1 -> Add/2
  uint2/1 -> Switch1/3
  Switch1/1 -> Unit Delay/1, GreaterOrEqual1/1
  Unit Delay/1 -> Add/1
  RollgCntrErrThd/1 -> DataTypeConversion2/1
  GreaterOrEqual1/1 -> RSLatch/1(S)
  Logical Operator1/1 -> RSLatch/2(R)
  RSLatch/1(Q) -> OR/1
  [RollgCntrOld] -> Subtract/2
  Subtract/1 -> Equal2/1
  uint4/1 -> Equal2/2
  [RollgCntrMax] -> Equal3/2
  UnitDelay3/1 -> [RollgCntrOld], Equal3/1
  Equal3/1 -> Switch3/2
  uint6/1 -> Equal4/2
  Equal4/1 -> Switch3/1
  Equal2/1 -> Switch3/3
  [RollgCntrOld] -> Equal1/2
  Switch3/1 -> Switch1/2
  Add/1 -> Switch1/1
  RollgCntr/1 -> DataTypeConversion/1
  DataTypeConversion1/1 -> [RollgCntrMax], Greater/2
  DataTypeConversion2/1 -> GreaterOrEqual1/2

== system ITKLib/Filter/GradientLimiter ==
  LU : Inport
  u : Inport  Port=2
  LL : Inport  Port=3
  dT : Inport  Port=4
  Delay : Delay  DelayLength=1  InitialConditionSource=Input port
      settings: InputPortMap=u0,p4
  MinMax1 : MinMax  Inputs=2  SaturateOnIntegerOverflow=on
  MinMax2 : MinMax  Inputs=2  SaturateOnIntegerOverflow=on
  MinMax3 : MinMax  Function=max  Inputs=2  SaturateOnIntegerOverflow=on
  MinMax4 : MinMax  Function=max  Inputs=2  SaturateOnIntegerOverflow=on
  Number1 : Constant  Value=0  OutDataTypeStr=single
      settings: AttributesFormatString=%<OutDataTypeStr>
  Number2 : Constant  Value=0  OutDataTypeStr=single
      settings: AttributesFormatString=%<OutDataTypeStr>
  Product : Product  Inputs=**  RndMeth=Zero  SaturateOnIntegerOverflow=on
  Product1 : Product  Inputs=**  RndMeth=Zero  SaturateOnIntegerOverflow=on
  Sum : Sum  SaturateOnIntegerOverflow=on
  Sum1 : Sum  Inputs=+-  SaturateOnIntegerOverflow=on
  y : Outport  InitialOutput=0
  wires:
  Sum/1 -> y/1, Delay/1
  u/1 -> [u], Sum1/1
  Delay/1 -> Sum/2, Sum1/2
  LL/1 -> Product1/1
  LU/1 -> Product/1
  MinMax1/1 -> MinMax3/1
  MinMax4/1 -> MinMax2/1
  dT/1 -> Product/2, Product1/2
  Sum1/1 -> MinMax3/2
  MinMax2/1 -> Sum/1
  MinMax3/1 -> MinMax2/2
  Number2/1 -> MinMax1/2
  Number1/1 -> MinMax4/2
  Product/1 -> MinMax4/1
  Product1/1 -> MinMax1/1
  [u] -> Delay/2

== system ITKLib/Filter/GradientLimiterRRV ==
  LU : Inport
  u : Inport  Port=2
  LL : Inport  Port=3
  E : Inport  Port=4
  R : Inport  Port=5  OutDataTypeStr=boolean
  RV : Inport  Port=6
  dT : Inport  Port=7
  Delay : Delay  DelayLength=1  InitialConditionSource=Input port
      settings: InputPortMap=u0,p4
  MinMax1 : MinMax  Inputs=2  SaturateOnIntegerOverflow=on
  MinMax2 : MinMax  Inputs=2  SaturateOnIntegerOverflow=on
  MinMax3 : MinMax  Function=max  Inputs=2  SaturateOnIntegerOverflow=on
  MinMax4 : MinMax  Function=max  Inputs=2  SaturateOnIntegerOverflow=on
  Number1 : Constant  Value=0  OutDataTypeStr=single
      settings: AttributesFormatString=%<OutDataTypeStr>
  Number2 : Constant  Value=0  OutDataTypeStr=single
      settings: AttributesFormatString=%<OutDataTypeStr>
  Product : Product  Inputs=**  RndMeth=Zero  SaturateOnIntegerOverflow=on
  Product1 : Product  Inputs=**  RndMeth=Zero  SaturateOnIntegerOverflow=on
  Sum : Sum  SaturateOnIntegerOverflow=on
  Sum1 : Sum  Inputs=+-  SaturateOnIntegerOverflow=on
  Switch1 : Switch  Criteria=u2 ~= 0  SaturateOnIntegerOverflow=off  InputSameDT=off
      settings: AttributesFormatString=Criteria : %<Criteria>
  Switch2 : Switch  Criteria=u2 ~= 0  InputSameDT=off
      settings: AttributesFormatString=Criteria : %<Criteria>
  Switch3 : Switch  Criteria=u2 ~= 0  InputSameDT=off
      settings: AttributesFormatString=Criteria : %<Criteria>
  y : Outport  InitialOutput=0
  wires:
  Product1/1 -> MinMax1/1
  Product/1 -> MinMax4/1
  Number1/1 -> MinMax4/2
  Number2/1 -> MinMax1/2
  MinMax3/1 -> MinMax2/2
  R/1 -> Switch1/2
  MinMax2/1 -> Sum/1
  Sum1/1 -> MinMax3/2
  dT/1 -> Product1/2, Product/2
  MinMax4/1 -> MinMax2/1
  MinMax1/1 -> MinMax3/1
  LU/1 -> Product/1
  LL/1 -> Product1/1
  RV/1 -> Switch1/1
  Switch3/1 -> Sum/2, Sum1/2
  u/1 -> Switch2/3, [u], Sum1/1
  E/1 -> Switch3/2, Switch2/2
  Switch2/1 -> y/1
  Sum/1 -> Switch1/3
  Switch1/1 -> Switch2/1, Delay/1
  Delay/1 -> Switch3/1
  [u] -> Switch3/3
  [u] -> Delay/2

== system ITKLib/Filter/GrdtAtFlgChg ==
  u : Inport
  TransFlg : Inport  Port=2
  Grdt : Inport  Port=3
  dT : Inport  Port=4
  Add1 : Sum
  DataTypeConversion : DataTypeConversion  OutDataTypeStr=int8  SaturateOnIntegerOverflow=off  RndMeth=Floor
  DataTypeConversion1 : DataTypeConversion  OutDataTypeStr=int8  SaturateOnIntegerOverflow=off  RndMeth=Floor
  EdgeRising1 : $bdroot/Memory/EdgeRising  Tag=initial value = 0
  FALSE : Constant  Description=FALSE  Value=0  OutDataTypeStr=boolean
      settings: AttributesFormatString=%<Description>
  Greater : RelationalOperator  Operator=>  OutDataTypeStr=boolean
  Logical Operator : Logic  AllPortsSameDT=off  OutDataTypeStr=boolean
  Logical Operator1 : Logic  Operator=NOT  AllPortsSameDT=off  OutDataTypeStr=boolean
  Logical Operator10 : Logic  Inputs=3  AllPortsSameDT=off  OutDataTypeStr=boolean
  Logical Operator11 : Logic  Operator=NOT  AllPortsSameDT=off  OutDataTypeStr=boolean
  Logical Operator4 : Logic  Operator=NOT  AllPortsSameDT=off  OutDataTypeStr=boolean
  Logical Operator7 : Logic  AllPortsSameDT=off  OutDataTypeStr=boolean
  Logical Operator9 : Logic  Operator=OR  AllPortsSameDT=off  OutDataTypeStr=boolean
  Max : MinMax  Function=max  Inputs=2  InputSameDT=on  SaturateOnIntegerOverflow=on
  Min : MinMax  Inputs=2  InputSameDT=on  SaturateOnIntegerOverflow=on
  Number2 : Constant  Value=0  OutDataTypeStr=single
      settings: AttributesFormatString=%<OutDataTypeStr>
  Number8 : Constant  Value=0  OutDataTypeStr=single
      settings: AttributesFormatString=%<OutDataTypeStr>
  Product : Product
  Product1 : Product
  RSLatch1 : $bdroot/Memory/RSLatch
  Relational Operator : RelationalOperator  Operator=~=  OutDataTypeStr=boolean  InputSameDT=off
  Sign : Signum
  Sign1 : Signum
  Subtract1 : Sum  Inputs=+-
  Subtract2 : Sum  Inputs=+-
  Switch{1..3,11..12} (5 alike) : Switch  Criteria=u2 ~= 0  SaturateOnIntegerOverflow=off  InputSameDT=off
      settings: AttributesFormatString=Criteria : %<Criteria>
  Unit Delay{2,5,8..9} (4 alike) : UnitDelay  SampleTime=-1  HasFrameUpgradeWarning=on
      Unit Delay2 settings: AttributesFormatString=<initial=%<x0>>
      Unit Delay5 settings: AttributesFormatString=<initial=%<X0>>
      Unit Delay8 settings: AttributesFormatString=<initial=%<X0>>
      Unit Delay9 settings: AttributesFormatString=<initial=%<X0>>
  TransOut : Outport
  TransEnd : Outport  Port=2
  TransActv : Outport  Port=3
  wires:
  Unit Delay9/1 -> Logical Operator9/2
  [TransEna] -> Logical Operator10/2
  Logical Operator9/1 -> Logical Operator10/3
  Relational Operator/1 -> Logical Operator9/1
  [TransEnd] -> Unit Delay8/1
  Logical Operator/1 -> Switch11/2
  [TransEna] -> Logical Operator/1
  Unit Delay8/1 -> Logical Operator4/1
  Logical Operator4/1 -> Logical Operator/2
  Switch11/1 -> Add1/2
  dT/1 -> Product/2
  RSLatch1/1 -> Switch1/2, [TransEna]  "TransEna"
  Number8/1 -> Switch11/3
  Product/1 -> Product1/2
  Switch12/1 -> Unit Delay2/1, TransOut/1
  [IniSign] -> DataTypeConversion/1
  Add1/1 -> Switch12/3, Subtract2/2
  Logical Operator10/1 -> Logical Operator11/1, [TransEnd], TransEnd/1, Unit Delay9/1, Switch12/2  "TransEnd"
  Subtract2/1 -> Sign1/1
  Sign1/1 -> DataTypeConversion1/1
  [TarVal] -> Subtract2/1, Switch12/1
  u/1 -> Switch1/3, Subtract1/1, [TarVal]  "TarVal"
  Sign/1 -> Greater/1, [IniSign], Product1/1  "IniSign"
  Grdt/1 -> Product/1
  [TransEna] -> Logical Operator7/2
  Logical Operator11/1 -> Logical Operator7/1
  Logical Operator7/1 -> TransActv/1  "TransActv"
  Unit Delay2/1 -> Switch1/1
  TransFlg/1 -> EdgeRising1/1, [TransFlg], RSLatch1/1
  Switch1/1 -> Subtract1/2, Add1/1  "TransInitVal"
  [TransEnd] -> Unit Delay5/1
  Unit Delay5/1 -> Switch3/3
  Product1/1 -> Min/2, Max/1  "TransVal"
  Number2/1 -> Greater/2
  Greater/1 -> Switch2/2
  Min/1 -> Switch2/1
  Max/1 -> Switch2/3
  Switch2/1 -> Switch11/1
  Subtract1/1 -> Sign/1, Min/1, Max/2
  DataTypeConversion/1 -> Relational Operator/1
  DataTypeConversion1/1 -> Relational Operator/2
  EdgeRising1/1 -> Switch3/2
  FALSE/1 -> Switch3/1
  Switch3/1 -> RSLatch1/2
  [TransFlg] -> Logical Operator1/1
  Logical Operator1/1 -> Logical Operator10/1

== system ITKLib/Filter/LowPass ==
  note: LP Filter y(n) = K*u(n) + (1-K)*y(n-1)
      | stability
      | 0 <= K=Ts/tau  <= 1
  T : Inport
  u : Inport  Port=2
  dT : Inport  Port=3
  Delay : Delay  DelayLength=1  InitialConditionSource=Input port
      settings: InputPortMap=u0,p4
  K : Product  Inputs=*/  SaturateOnIntegerOverflow=on
  MinMax : MinMax  Function=max  Inputs=3  SaturateOnIntegerOverflow=on
  Product : Product  RndMeth=Zero  SaturateOnIntegerOverflow=on
  Subtract : Sum  SaturateOnIntegerOverflow=on
  dif : Sum  Inputs=+-  SaturateOnIntegerOverflow=on
  single : Constant  Value=0.00001  OutDataTypeStr=single  SampleTime=-1
      settings: AttributesFormatString=%<OutDataTypeStr>
  y : Outport
  wires:
  u/1 -> [u], dif/1
  dif/1 -> Product/2
  Delay/1 -> Subtract/2, dif/2
  K/1 -> Product/1
  Product/1 -> Subtract/1
  MinMax/1 -> K/2
  T/1 -> MinMax/2
  dT/1 -> K/1, MinMax/1
  Subtract/1 -> Delay/1, y/1
  [u] -> Delay/2
  single/1 -> MinMax/3

== system ITKLib/Filter/LowPassERRV ==
  note: LP Filter y(n) = K*u(n) + (1-K)*y(n-1)
      | stability
      | 0 <= K=Ts/tau  <= 1
  T : Inport
  u : Inport  Port=2
  E : Inport  Port=3
  R : Inport  Port=4
  RV : Inport  Port=5
  dT : Inport  Port=6
  Delay : Delay  DelayLength=1  InitialConditionSource=Input port
      settings: InputPortMap=u0,p4
  K : Product  Inputs=*/  SaturateOnIntegerOverflow=on
  MinMax1 : MinMax  Function=max  Inputs=3  SaturateOnIntegerOverflow=on
  Product : Product  RndMeth=Zero  SaturateOnIntegerOverflow=on
  Subtract : Sum  SaturateOnIntegerOverflow=on
  Switch1 : Switch  Criteria=u2 ~= 0  InputSameDT=off
      settings: AttributesFormatString=Criteria : %<Criteria>
  Switch2 : Switch  Criteria=u2 ~= 0  InputSameDT=off
      settings: AttributesFormatString=Criteria : %<Criteria>
  Switch3 : Switch  Criteria=u2 ~= 0  InputSameDT=off
      settings: AttributesFormatString=Criteria : %<Criteria>
  dif : Sum  Inputs=+-  SaturateOnIntegerOverflow=on
  single : Constant  Value=0.00001  OutDataTypeStr=single  SampleTime=-1
      settings: AttributesFormatString=%<OutDataTypeStr>
  y : Outport
  wires:
  R/1 -> Switch2/2
  Subtract/1 -> Switch2/3
  Switch2/1 -> Delay/1, Switch1/1
  dT/1 -> MinMax1/1, K/1
  dif/1 -> Product/2
  T/1 -> MinMax1/2
  Product/1 -> Subtract/1
  MinMax1/1 -> K/2
  E/1 -> Switch3/2, Switch1/2
  Switch1/1 -> y/1
  K/1 -> Product/1
  u/1 -> [u], Switch1/3, dif/1
  RV/1 -> Switch2/1
  Switch3/1 -> dif/2, Subtract/2
  Delay/1 -> Switch3/1
  [u] -> Switch3/3
  [u] -> Delay/2
  single/1 -> MinMax1/3

== system ITKLib/Filter/LowPassFrq ==
  u : Inport
  Frq : Inport  Port=2
  dT : Inport  Port=3
  Divide : Product  Inputs=*/  InputSameDT=on  SaturateOnIntegerOverflow=on
  LowPass : $bdroot/Filter/LowPass
  Math Function : Math
  Max : MinMax  Function=max  Inputs=2  InputSameDT=on  SaturateOnIntegerOverflow=on
  Max1 : MinMax  Function=max  Inputs=2  InputSameDT=on  SaturateOnIntegerOverflow=on
  Opposite : $bdroot/BasicOperators/Opposite
  Product1 : Product  InputSameDT=on  SaturateOnIntegerOverflow=on
  Product2 : Product  Inputs=3  RndMeth=Zero  SaturateOnIntegerOverflow=on
  Subtract1 : Sum  Inputs=+-  InputSameDT=on  SaturateOnIntegerOverflow=on
  single1 : Constant  Value=0.0000001  OutDataTypeStr=single  SampleTime=-1
      settings: AttributesFormatString=%<OutDataTypeStr>
  single2 : Constant  Value=3.1415926  OutDataTypeStr=single  SampleTime=-1
      settings: AttributesFormatString=%<OutDataTypeStr>
  single3 : Constant  Value=2  OutDataTypeStr=single  SampleTime=-1
      settings: AttributesFormatString=%<OutDataTypeStr>
  single4 : Constant  OutDataTypeStr=single  SampleTime=-1
      settings: AttributesFormatString=%<OutDataTypeStr>
  y : Outport
  wires:
  Product1/1 -> Math Function/1
  single1/1 -> Max/2
  Max1/1 -> LowPass/1
  Math Function/1 -> Subtract1/2
  u/1 -> LowPass/2
  Frq/1 -> Product2/1
  Divide/1 -> Max1/2
  Opposite/1 -> Product1/1
  Max/1 -> Divide/2
  dT/1 -> Max1/1, Divide/1, Product1/2, LowPass/3
  Subtract1/1 -> Max/1
  single4/1 -> Subtract1/1
  LowPass/1 -> y/1
  single2/1 -> Product2/2
  Product2/1 -> Opposite/1
  single3/1 -> Product2/3

== system ITKLib/Filter/LowPassFrqERRV ==
  note: LP Filter y(n) = K*u(n) + (1-K)*y(n-1)
      | stability
      | 0 <= K=Ts/tau  <= 1
  u : Inport
  Frq : Inport  Port=2
  E : Inport  Port=3
  R : Inport  Port=4
  RV : Inport  Port=5
  Delay : Delay  DelayLength=1  InitialConditionSource=Input port
      settings: InputPortMap=u0,p4
  Product : Product  RndMeth=Zero  SaturateOnIntegerOverflow=on
  Subtract : Sum  SaturateOnIntegerOverflow=on
  Switch1 : Switch  Criteria=u2 ~= 0  InputSameDT=off
      settings: AttributesFormatString=Criteria : %<Criteria>
  Switch2 : Switch  Criteria=u2 ~= 0  InputSameDT=off
      settings: AttributesFormatString=Criteria : %<Criteria>
  Switch3 : Switch  Criteria=u2 ~= 0  InputSameDT=off
      settings: AttributesFormatString=Criteria : %<Criteria>
  dif : Sum  Inputs=+-  SaturateOnIntegerOverflow=on
  y : Outport
  wires:
  [u] -> Delay/2
  [u] -> Switch3/3
  Delay/1 -> Switch3/1
  Switch3/1 -> dif/2, Subtract/2
  RV/1 -> Switch2/1
  u/1 -> dif/1, Switch1/3, [u]
  Frq/1 -> Product/1
  Switch1/1 -> y/1
  E/1 -> Switch1/2, Switch3/2
  Product/1 -> Subtract/1
  dif/1 -> Product/2
  Switch2/1 -> Switch1/1, Delay/1
  Subtract/1 -> Switch2/3
  R/1 -> Switch2/2

== system ITKLib/Filter/MoveAvrgFilt ==
  note: [m]
  note: [ws/m]
  note: [ws]
  note: [m]
  note: [m]
  note: [ws]
  oldY : Inport
  filCon : Inport  Port=2
  deltaStep : Inport  Port=3
  in : Inport  Port=4
  max : Inport  Port=5
  min : Inport  Port=6
  fldPrms : Inport  Port=7
  Add : Sum  RndMeth=Simplest  SaturateOnIntegerOverflow=on
  Divide : Product  Inputs=*/  RndMeth=Simplest  SaturateOnIntegerOverflow=on
  Limit1 : Subsystem  Description=""  RTWFcnName=Limit  RTWFileName=BoschITK_Mdl_Lib  mask(LimitWoFlag){}
      mask help:
      | Limits the input value u between the maximum (MX) and the minimum (MN) values.
      |
      | The input value u is checked first against the minimum value and then against the maximum value.
      |
      | In addition to that a flag is set in case the current value is higher than MX and another flag is set in case the current value is smaller than the MN value.
      |
      | inputs:
      | MX  - maximum allowed value
      | MN  - minimal allowed value
      | u   - input value to be evaluated
      |
      | outputs:
      | y       - limited output value
      |
      | Simulink Custom Model Library, created by MCC.
      settings: RTWFcnNameOpts=User specified  RTWFileNameOpts=User specified
      mask Display:
      | color('black');
      | plot([0.2,0.8],[0.5,0.5]);
      | plot([0.5,0.5],[0.2,0.8]);
      | plot([0.75,0.8,0.75],[0.53,0.5,0.47]);
      | plot([0.53,0.5,0.47],[0.75,0.8,0.75]);
      | color('red');
      | plot([0.2,0.3,0.7,0.8],[0.3,0.3,0.7,0.7]);
      | color('green');
      | text(1,0,'ITK','horizontalAlignment','right','verticalAlignment','bottom');
  Product1 : Product  RndMeth=Simplest  SaturateOnIntegerOverflow=on
  Product2 : Product  RndMeth=Simplest  SaturateOnIntegerOverflow=on
  Subtract : Sum  Inputs=+-  RndMeth=Simplest  SaturateOnIntegerOverflow=on
  Switch : Switch  Criteria=u2 ~= 0  RndMeth=Simplest  InputSameDT=off
      settings: AttributesFormatString=%<Criteria>\nThreshold:%<Threshold>
  y : Outport
  wires:
  fldPrms/1 -> Switch/2
  Divide/1 -> Limit1/2(u)
  Product2/1 -> Add/2
  Limit1/1(y) -> Switch/1
  min/1 -> Limit1/3(MN)
  filCon/1 -> Divide/2, Subtract/1
  deltaStep/1 -> Subtract/2, Product2/1
  max/1 -> Limit1/1(MX)
  oldY/1 -> Switch/3, Product1/1
  Subtract/1 -> Product1/2
  Add/1 -> Divide/1
  Product1/1 -> Add/1
  Switch/1 -> y/1
  in/1 -> Product2/2

== system ITKLib/Filter/RampLimiter ==
  In : Inport
  LimitUp : Inport  Port=2
  LimitDown : Inport  Port=3
  Enable : Inport  Port=4
  Add : Sum  Inputs=+-  OutDataTypeStr=single  SaturateOnIntegerOverflow=on
  Add1 : Sum  OutDataTypeStr=single  SaturateOnIntegerOverflow=on
  Add2 : Sum  Inputs=+-  OutDataTypeStr=single  SaturateOnIntegerOverflow=on
  Add3 : Sum  Inputs=+-  OutDataTypeStr=single  SaturateOnIntegerOverflow=on
  Constant1 : Constant  Value=0  OutDataTypeStr=uint8  SampleTime=-1
  Constant2 : Constant  Value=0  OutDataTypeStr=uint8  SampleTime=-1
  Data Type Conversion : DataTypeConversion  OutDataTypeStr=single  SaturateOnIntegerOverflow=off  RndMeth=Floor
  Data Type Conversion1 : DataTypeConversion  OutDataTypeStr=single  SaturateOnIntegerOverflow=off  RndMeth=Floor
  Data Type Conversion2 : DataTypeConversion  OutDataTypeStr=single  SaturateOnIntegerOverflow=off  RndMeth=Floor
  Logical Operator1 : Logic  AllPortsSameDT=off  OutDataTypeStr=boolean
  Logical Operator2 : Logic  AllPortsSameDT=off  OutDataTypeStr=boolean
  Relational Operator{,2..5} (5 alike) : RelationalOperator  Operator=>  OutDataTypeStr=boolean  InputSameDT=off
  Switch{1..4} (4 alike) : Switch  Criteria=u2 ~= 0  OutDataTypeStr=single  InputSameDT=off
  Unit Delay : UnitDelay  SampleTime=-1  HasFrameUpgradeWarning=on
  Out : Outport  VectorParamsAs1DForOutWhenUnconnected=off
  wires:
  Add/1 -> Relational Operator2/1, Relational Operator/1
  Relational Operator3/1 -> Logical Operator2/1
  Relational Operator4/1 -> Logical Operator2/2
  Relational Operator2/1 -> Logical Operator1/2
  Switch1/1 -> Switch4/1
  Add1/1 -> Switch2/1
  Unit Delay/1 -> Relational Operator5/2, Add2/1, Add3/1, Add/2, Add1/2
  LimitDown/1 -> Data Type Conversion2/1
  Switch2/1 -> Switch1/1
  Add2/1 -> Relational Operator4/1, Relational Operator3/1
  Logical Operator1/1 -> Switch2/2
  Enable/1 -> Switch4/2
  Relational Operator5/1 -> Switch1/2
  In/1 -> Data Type Conversion/1
  Constant2/1 -> Relational Operator4/2
  Switch3/1 -> Switch1/3
  Data Type Conversion2/1 -> Add3/2, Relational Operator3/2
  LimitUp/1 -> Data Type Conversion1/1
  Relational Operator/1 -> Logical Operator1/1
  Constant1/1 -> Relational Operator2/2
  Switch4/1 -> Unit Delay/1, Out/1
  Data Type Conversion/1 -> Switch4/3, Relational Operator5/1, Switch3/3, Add2/2, Switch2/3, Add/1
  Data Type Conversion1/1 -> Add1/1, Relational Operator/2
  Logical Operator2/1 -> Switch3/2
  Add3/1 -> Switch3/1
